simulink model "ResonantLLCConverter"  (R2020b)
settings: Solver=VariableStepAuto  StartTime=0.0  StopTime=0.002  MaxStep=1e-4  RelTol=1e-4  EnableMultiTasking=on
PreLoadFcn:
  | Rs_fet=1e8;  % FET snubber resistance (ohms)
  | Cs_fet=inf;  % FET snubber capacitance (ohms)
  | Vf=0.6;        % Diode forward voltage (V)
libraries: powerlib x18, powerlib_meascontrol x2
Description:
  | Copyright 2008-2019 The MathWorks, Inc.
settings Model: SimulationMode=accelerator  Creator=MathWorks  LastModifiedBy=lauramarks2
settings SolverCC: SolverResetMethod=Robust
settings OptimizationCC: LifeSpan=inf
settings DebuggingCC: ReadBeforeWriteMsg=DisableAll  WriteAfterWriteMsg=DisableAll  WriteAfterReadMsg=DisableAll  MultiTaskDSMMsg=none  SFUnexpectedBacktrackingDiag=warning  SFNoUnconditionalDefaultTransitionDiag=warning  SFExecutionAtInitializationDiag=none  ArithmeticOperatorsInVariantConditions=warning
settings ModelReferenceCC: UpdateModelReferenceTargets=IfOutOfDate
settings SFSimCC: SFSimEcho=off  SimUseLocalCustomCode=off  CustomCodeUndefinedFunction=UseInterfaceOnly
settings RTWCC: RTWUseLocalCustomCode=off
settings CodeAppCC: StateflowObjectComments=on
settings GRTTargetCC: TargetLangStandard=C89/C90 (ANSI)
settings ConfigComp: CovMetricSettings=dw  CovSaveCumulativeToWorkspaceVar=on  CovSaveSingleToWorkspaceVar=on  CovExternalEMLEnable=off
settings SimscapeCC: SimscapeNormalizeSystem=off  SimscapeNominalValues={1, 'bar'; 1, 'cm^3/s'; 1, 'bar*kg/s'; 1, 'kJ/kg'; 1, 'kW'; }

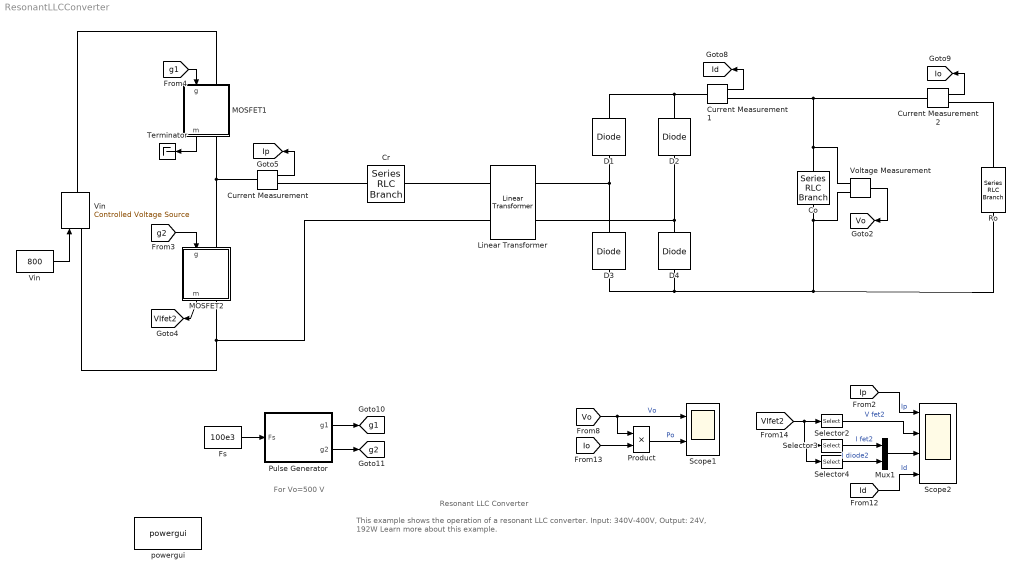
== system ResonantLLCConverter ==
  note: For Vo=500 V
  note: Resonant LLC Converter
  note: This example shows the operation of a resonant LLC converter.
      | Input: 340V-400V, Output: 24V, 192W
      |
      | Learn more about this example.
  Co : powerlib/Elements/Series RLC Branch  LConnTagsString=__new0  RConnTagsString=__new0  BranchType=C  Resistance=1e-4  Inductance=200e-6  SetiL0=off  InitialCurrent=0  Capacitance=100e-6  Setx0=on  InitialVoltage=24  Measurements=None
  Cr : powerlib/Elements/Series RLC Branch  LConnTagsString=__new0  RConnTagsString=__new0  BranchType=C  Resistance=1e-4  Inductance=200e-6  SetiL0=off  InitialCurrent=0  Capacitance=15e-9  Setx0=off  InitialVoltage=40  Measurements=None
  Current Measurement : powerlib/Measurements/Current Measurement  PhasorSimulation=off  OutputType=Complex  PSBequivalent=0
  Current Measurement1 : powerlib/Measurements/Current Measurement  PhasorSimulation=off  OutputType=Complex  PSBequivalent=0
  Current Measurement2 : powerlib/Measurements/Current Measurement  PhasorSimulation=off  OutputType=Complex  PSBequivalent=0
  D{1..4} (4 alike) : powerlib/Power Electronics/Diode  Ron=1e-3  Lon=0  Vf=0.5  IC=0  UseSnubber=off  Rs=1e6  Cs=inf  Measurements=off
  Fs : Constant  Value=100e3
  Linear Transformer : powerlib/Elements/Linear Transformer  UNITS=SI  NominalPower=[ 200 85e3 ]  winding1="[52   1e-2  102e-6]"  winding2="[6  1e-2  1.36e-6 ]"  ThreeWindings=off  winding3=[3.15e+05 0.7938 0.084225]  RmLm=[1e4 963e-6]  Measurements=None  DataType=on
  MOSFET1 : Subsystem
  MOSFET2 : Subsystem
  Mux1 : Mux  Inputs=2
  Product : Product
  Pulse Generator : Subsystem
  Ro : powerlib/Elements/Series RLC Branch  LConnTagsString=__new0  RConnTagsString=__new0  BranchType=R  Resistance=5  Inductance=200e-6  SetiL0=off  InitialCurrent=0  Capacitance=400e-6  Setx0=off  InitialVoltage=0  Measurements=None
  Scope1 : Scope  NumInputPorts=2
  Scope2 : Scope  NumInputPorts=4
  Selector2 : Selector  InputPortWidth=3  IndexOptions=Index vector (dialog)  Indices=2  OutputSizes=1
  Selector3 : Selector  InputPortWidth=3  IndexOptions=Index vector (dialog)  Indices=1  OutputSizes=1
  Selector4 : Selector  InputPortWidth=3  IndexOptions=Index vector (dialog)  Indices=3  OutputSizes=1
  Terminator : Terminator
  Vin : Constant  Value=800
  "Vin " : powerlib/Electrical Sources/Controlled Voltage Source  Initialize=on  Source_Type=DC  Amplitude=0  Phase=0  Frequency=0  Measurements=None
  Voltage Measurement : powerlib/Measurements/Voltage Measurement  PhasorSimulation=off  OutputType=Complex  PSBequivalent=0
  powergui : powerlib/powergui  Priority=1  SimulationMode=Continuous  SampleTime=50e-6  frequency=60  Iterations=50  frequencyindice=0  Pbase=100e6  ErrMax=1e-4  UnitsV=kV  UnitsW=MW  buscounter=0  FunctionMessages=off  echomessages=off  EnableUseOfTLC=off  CurrentSourceSwitches=off  DisableSnubberDevices=off  DisableRonSwitches=off  DisableVfSwitches=off  DisplayEquations=off  AutomaticDiscreteSolvers=off  SolverType=Tustin/Backward Euler (TBE)  Interpol=off  ExternalGateDelay=off  methode=off  Ts=10  x0status=blocks  SPID=on  SwTol=0  HookPort=off  NonlinearTolerance=0  nMaxIteration=15  ContinueOnMaxIteration=off  RestoreLinks=warning  ResistiveCurrentMeasurement=off  Frange=[0:2:500]  Ylog=off  Xlog=on  ShowGrid=off  save=off  variable=ZData  structure=0  ZoomFFT=off  StartTime=0.0  cycles=1  DisplayStyle=1  fundamental=60  FreqAxis=off  MaxFrequency=1000  frequencyindicesteady=1  RmsSteady=1  display=off
  tag scope: Id=global, Io=global, Ip=global, VIfet2=global, Vo=global, g1=global, g2=global
  wires:
  [g2] -> MOSFET2/1(g)
  [g1] -> MOSFET1/1(g)
  MOSFET1/1(m) -> Terminator/1
  Current Measurement/1 -> [Ip]
  Voltage Measurement/1 -> [Vo]
  Current Measurement1/1 -> [Id]
  Current Measurement2/1 -> [Io]
  [Io] -> Product/2
  Pulse Generator/1(g1) -> [g1]
  Pulse Generator/2(g2) -> [g2]
  Fs/1 -> Pulse Generator/1(Fs)
  Product/1 -> Scope1/2  "Po"
  [Vo] -> Product/1, Scope1/1  "Vo"
  MOSFET2/1(m) -> [VIfet2]
  Vin/1 -> "Vin "/1
  [Id] -> Scope2/4  "Id"
  [Ip] -> Scope2/1  "Ip"
  Selector3/1 -> Mux1/1  "I fet2"
  Selector2/1 -> Scope2/2  "V fet2"
  Mux1/1 -> Scope2/3
  Selector4/1 -> Mux1/2  "I diode2"
  [VIfet2] -> Selector4/1, Selector3/1, Selector2/1
  connections:
  Co/RConn1 -- Voltage Measurement/LConn2 -- Ro/RConn1 -- D4/LConn1 -- D3/LConn1
  Linear Transformer/RConn1 -- D1/LConn1 -- D3/RConn1
  Current Measurement/LConn1 -- MOSFET2/LConn1 -- MOSFET1/RConn1
  Linear Transformer/RConn2 -- D2/LConn1 -- D4/RConn1
  MOSFET1/LConn1 -- "Vin "/RConn1
  "Vin "/LConn1 -- Linear Transformer/LConn2 -- MOSFET2/RConn1
  Cr/LConn1 -- Current Measurement/RConn1
  D1/RConn1 -- D2/RConn1 -- Current Measurement1/LConn1
  Voltage Measurement/LConn1 -- Current Measurement2/LConn1 -- Current Measurement1/RConn1 -- Co/LConn1
  Current Measurement2/RConn1 -- Ro/LConn1
  Linear Transformer/LConn1 -- Cr/RConn1

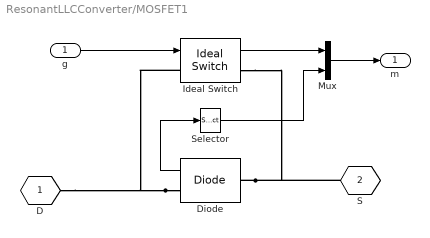
== system ResonantLLCConverter/MOSFET1 ==
  g : Inport
  Diode : powerlib/Power Electronics/Diode  Ron=1e-3  Lon=0  Vf=Vf  IC=0  UseSnubber=0  Rs=inf  Cs=0  Measurements=on
  Ideal Switch : powerlib/Power Electronics/Ideal Switch  Ron=1e-3  Lon=0  IC=0  Rs=Rs_fet  Cs=Cs_fet  Measurements=on
  Mux : Mux  Inputs=[2,1]
  Selector : Selector  InputPortWidth=2  IndexOptions=Index vector (dialog)  Indices=1  OutputSizes=1
  D : PMIOPort  Tag=PMCPort  Side=Left
  S : PMIOPort  Tag=PMCPort  Port=2  Side=Right
  m : Outport  VectorParamsAs1DForOutWhenUnconnected=off
  wires:
  Diode/1 -> Selector/1
  g/1 -> Ideal Switch/1
  Ideal Switch/1 -> Mux/1
  Selector/1 -> Mux/2
  Mux/1 -> m/1
  connections:
  Diode/LConn1 -- S/RConn1 -- Ideal Switch/RConn1
  Diode/RConn1 -- D/RConn1 -- Ideal Switch/LConn1

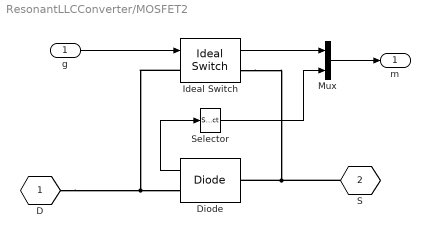
== system ResonantLLCConverter/MOSFET2 ==
  g : Inport
  Diode : powerlib/Power Electronics/Diode  Ron=1e-3  Lon=0  Vf=Vf  IC=0  UseSnubber=0  Rs=inf  Cs=0  Measurements=on
  Ideal Switch : powerlib/Power Electronics/Ideal Switch  Ron=1e-3  Lon=0  IC=0  Rs=Rs_fet  Cs=Cs_fet  Measurements=on
  Mux : Mux  Inputs=[2,1]
  Selector : Selector  InputPortWidth=2  IndexOptions=Index vector (dialog)  Indices=1  OutputSizes=1
  D : PMIOPort  Tag=PMCPort  Side=Left
  S : PMIOPort  Tag=PMCPort  Port=2  Side=Right
  m : Outport  VectorParamsAs1DForOutWhenUnconnected=off
  wires:
  Mux/1 -> m/1
  Selector/1 -> Mux/2
  Ideal Switch/1 -> Mux/1
  g/1 -> Ideal Switch/1
  Diode/1 -> Selector/1
  connections:
  Ideal Switch/LConn1 -- D/RConn1 -- Diode/RConn1
  Ideal Switch/RConn1 -- S/RConn1 -- Diode/LConn1

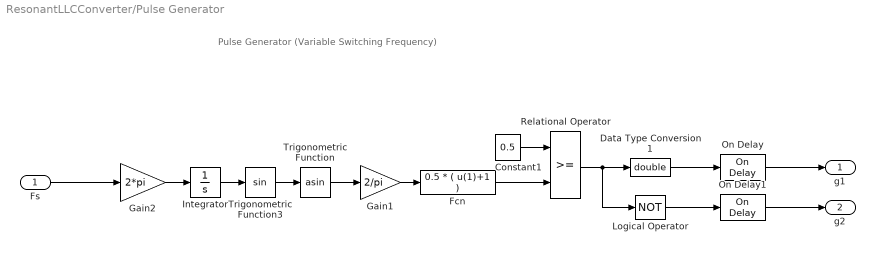
== system ResonantLLCConverter/Pulse Generator ==
  note: Pulse Generator
      | (Variable Switching Frequency)
  Fs : Inport
  Constant1 : Constant  Value=0.5
  Data Type Conversion1 : DataTypeConversion  OutDataTypeStr=double
  Fcn : Fcn  Expr=0.5 * ( u(1)+1 )
  Gain1 : Gain  Gain=2/pi  SaturateOnIntegerOverflow=on  OutDataTypeStr=Inherit: Same as input  ParamDataTypeStr=Inherit: Same as input
  Gain2 : Gain  Gain=2*pi  SaturateOnIntegerOverflow=on  OutDataTypeStr=Inherit: Same as input  ParamDataTypeStr=Inherit: Same as input
  Integrator : Integrator
  Logical Operator : Logic  Operator=NOT  AllPortsSameDT=off  OutDataTypeStr=float('double')
  On Delay : powerlib_meascontrol/Logic/On Delay  DelayType=On delay  delay=400e-9  ic=0  Ts=0
  On Delay1 : powerlib_meascontrol/Logic/On Delay  DelayType=On delay  delay=400e-9  ic=0  Ts=0
  Relational Operator : RelationalOperator  OutDataTypeStr=boolean  RndMeth=Nearest
  Trigonometric Function : Trigonometry  Operator=asin
  Trigonometric Function3 : Trigonometry
  g1 : Outport  VectorParamsAs1DForOutWhenUnconnected=off
  g2 : Outport  Port=2  VectorParamsAs1DForOutWhenUnconnected=off
  wires:
  Trigonometric Function3/1 -> Trigonometric Function/1
  Gain1/1 -> Fcn/1
  Trigonometric Function/1 -> Gain1/1
  Integrator/1 -> Trigonometric Function3/1
  Constant1/1 -> Relational Operator/1
  Relational Operator/1 -> Data Type Conversion1/1, Logical Operator/1
  Fcn/1 -> Relational Operator/2
  Logical Operator/1 -> On Delay1/1
  Data Type Conversion1/1 -> On Delay/1
  Gain2/1 -> Integrator/1
  Fs/1 -> Gain2/1
  On Delay/1 -> g1/1
  On Delay1/1 -> g2/1
